simulink model "ModelReferencing2"  (R2021a)
settings: Solver=VariableStepAuto  StartTime=0.0  StopTime=10.0  RelTol=1e-3
settings Model: Creator=20204920  LastModifiedBy=20204920

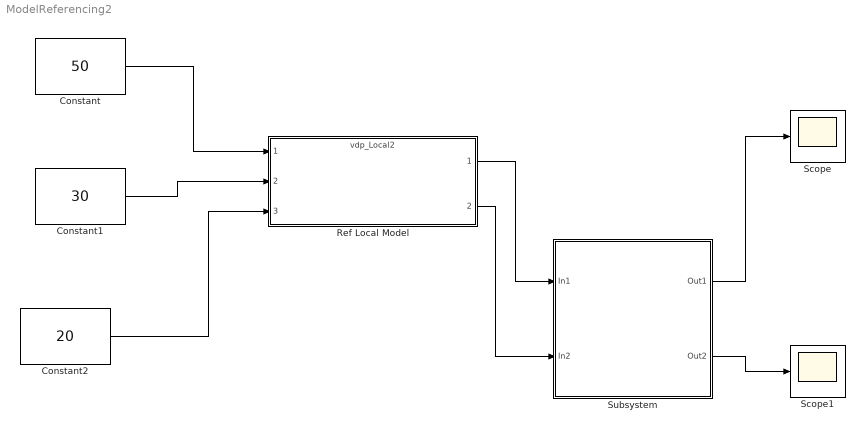
== system ModelReferencing2 ==
  Constant : Constant  Value=50
  Constant1 : Constant  Value=30
  Constant2 : Constant  Value=20
  Ref Local Model : ModelReference  ModelNameDialog=vdp_Local2.slx  SimulationMode=Normal  ModelReferenceVersion=1.3
  Scope : Scope
  Scope1 : Scope
  Subsystem : Subsystem
  wires:
  Constant/1 -> Ref Local Model/1
  Constant1/1 -> Ref Local Model/2
  Subsystem/1(Out1) -> Scope/1
  Subsystem/2(Out2) -> Scope1/1
  Constant2/1 -> Ref Local Model/3
  Ref Local Model/1 -> Subsystem/1(In1)
  Ref Local Model/2 -> Subsystem/2(In2)

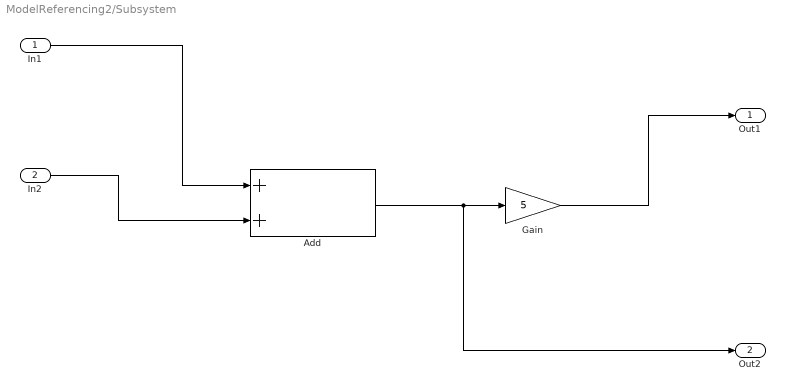
== system ModelReferencing2/Subsystem ==
  In1 : Inport
  In2 : Inport  Port=2
  Add : Sum
  Gain : Gain  Gain=5
  Out1 : Outport
  Out2 : Outport  Port=2
  wires:
  Add/1 -> Out2/1, Gain/1
  In1/1 -> Add/1
  Gain/1 -> Out1/1
  In2/1 -> Add/2
